simulink model "servotestin"  (R2020b)
settings: Solver=VariableStepAuto  StartTime=0.0  StopTime=10.0  RelTol=1e-3
model workspace (MAT data in the model file):
  BACKLASH_DEADBAND_RAD = Simulink.Parameter
  BACKLASH_DEADBAND_RAD.Value = 0.349065850399
  BACKLASH_DEADBAND_RAD.DataType = 'auto'
  BACKLASH_DEADBAND_RAD.Dimensions = [1 1]
  LEG_INERTIA = Simulink.Parameter
  LEG_INERTIA.Value = 0.01
  LEG_INERTIA.DataType = 'auto'
  LEG_INERTIA.Dimensions = [1 1]
libraries: fl_lib x7, nesl_utility x5, ee_lib x3, simulink_extras x2
settings Model: OrderedModelArguments=off  Creator=Adam  LastModifiedBy=Adam

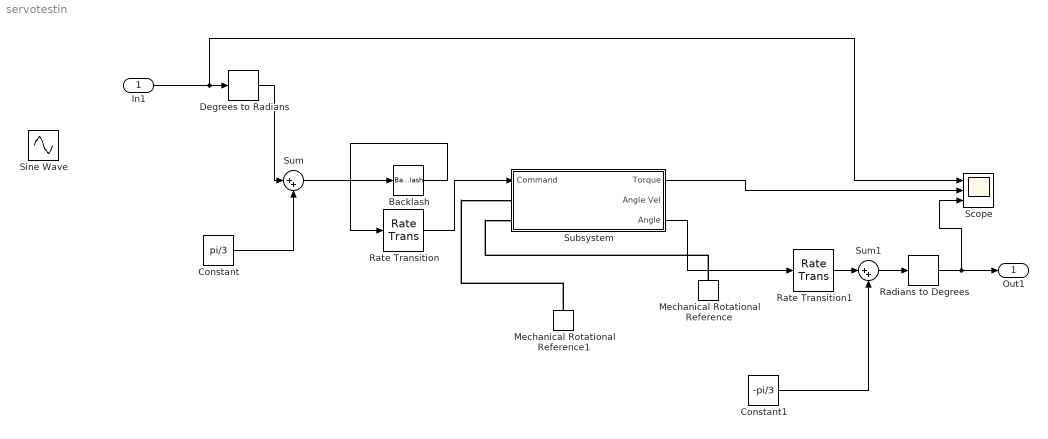
== system servotestin ==
  In1 : Inport
  Backlash : Backlash  BacklashWidth=BACKLASH_DEADBAND_RAD_M  InitialOutput=pi / 3
  Constant : Constant  Value=pi/3
  Constant1 : Constant  Value=-pi/3
  Degrees to Radians : simulink_extras/Transformations/Degrees to Radians
  Mechanical Rotational Reference : fl_lib/Mechanical/Rotational Elements/Mechanical Rotational Reference
  Mechanical Rotational Reference1 : fl_lib/Mechanical/Rotational Elements/Mechanical Rotational Reference
  Radians to Degrees : simulink_extras/Transformations/Radians to Degrees
  Rate Transition : RateTransition  InitialCondition=pi/3  OutPortSampleTime=1/330
  Rate Transition1 : RateTransition  InitialCondition=pi/3  OutPortSampleTime=.015
  Scope : Scope  NumInputPorts=3
  Sine Wave : Sin  Amplitude=20  Frequency=16  SampleTime=0
  Subsystem : Subsystem
  Sum : Sum  Inputs=|++
  Sum1 : Sum  Inputs=|++
  Out1 : Outport
  wires:
  In1/1 -> Scope/1, Degrees to Radians/1
  Subsystem/3(Angle) -> Rate Transition1/1
  Constant/1 -> Sum/2
  Sum/1 -> Backlash/1
  Rate Transition/1 -> Subsystem/1(Command)
  Subsystem/1(Torque) -> Scope/2
  Backlash/1 -> Rate Transition/1
  Degrees to Radians/1 -> Sum/1
  Radians to Degrees/1 -> Scope/3, Out1/1
  Constant1/1 -> Sum1/2
  Sum1/1 -> Radians to Degrees/1
  Rate Transition1/1 -> Sum1/1
  connections:
  Mechanical Rotational Reference1/LConn1 -- Subsystem/LConn1
  Mechanical Rotational Reference/LConn1 -- Subsystem/LConn2

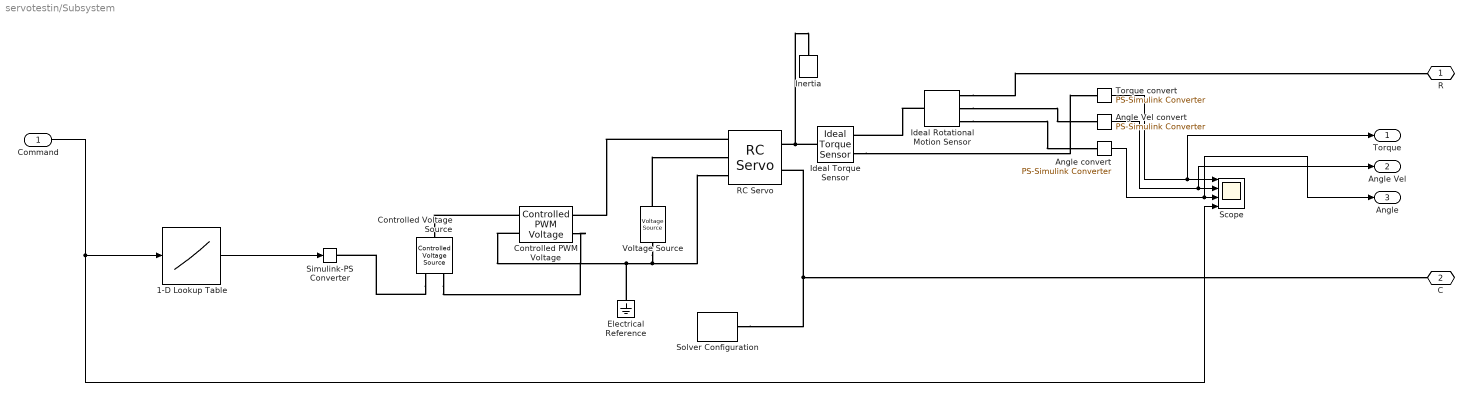
== system servotestin/Subsystem ==
  Command : Inport
  1-D Lookup Table : Lookup_n-D  NumberOfTableDimensions=1  BreakpointsForDimension1=[0 2*pi/3]  Table=[1.485 3.465]  InternalRulePriority=Speed  RndMeth=Simplest  InputSameDT=on
  Angle Vel convert : nesl_utility/PS-Simulink Converter  PhysicalDomain=network_engine_domain  SubClassName=ps_output  LeftPortType=input  RightPortType=output  PseudoPeriodic=off  Frequencies=[]  Unit=inherit  AffineConversion=off
  Angle convert : nesl_utility/PS-Simulink Converter  PhysicalDomain=network_engine_domain  SubClassName=ps_output  LeftPortType=input  RightPortType=output  PseudoPeriodic=off  Frequencies=[]  Unit=inherit  AffineConversion=off
  Controlled PWM Voltage : ee_lib/Integrated Circuits/Controlled PWM Voltage  F=330 Hz  TD=0 s  pulse_width_offset=0 s  pulse_min=0 s  Vmin=0 V  Vmax=5 V  Vm=5 V  pwm_or_av=1  event_type=1  sample_time=1e-6 s  u_min=0  u_max=1
  Controlled Voltage Source : fl_lib/Electrical/Electrical Sources/Controlled Voltage Source
  Electrical Reference : fl_lib/Electrical/Electrical Elements/Electrical Reference
  Ideal Rotational Motion Sensor : fl_lib/Mechanical/Mechanical Sensors/Ideal Rotational Motion Sensor  wrap_angle=simscape.enum.onoff.off  offset=60 deg
  Ideal Torque Sensor : fl_lib/Mechanical/Mechanical Sensors/Ideal Torque Sensor
  Inertia : fl_lib/Mechanical/Rotational Elements/Inertia  inertia=LEG_INERTIA_M kg*m^2  num_ports=foundation.enum.numPorts2.one  w_specify=off  w_priority=High  w=0 rad/s  w_nominal_specify=off  w_nominal_unit=rad/s  w_nominal_value=1  t_specify=off  t_priority=None  t=0 N*m  t_nominal_specify=off  t_nominal_unit=N*m  t_nominal_value=1
  RC Servo : ee_lib/Electromechanical/Brushed Motors/RC Servo  stall_torque=35 kg*cm  time_60=.11 s  nominal_voltage=7.2 V  rotational_range=[0, 120] deg  pulse_width_range=[900, 2100] us  threshold=3 V  R_s=18 kOhm  resolution=0.2 deg  angle_meas_error=0 deg  backdrive_torque=0.5 kg*cm  ratio=320  inertia=0.01 g*cm^2  endstop_angles=[-5, 185] deg  endstop_stiffness=1e6 N*m/rad  endstop_damping=0.01 N*m/(rad/s)  enable_faults=0  fault_action=1  fault_type=1  enable_temporal_fault=0  t_fault=1 s  enable_behavioral_fault=0  max_permissible_current=1 A  t_fail_on_current=1 s  angle_specify=on  angle_priority=High  angle=60 deg  angle_nominal_specify=off  angle_nominal_unit=deg  angle_nominal_value=1  w_specify=off  w_priority=High  w=0 deg/s  w_nominal_specify=off  w_nominal_unit=deg/s  w_nominal_value=1  torque_specify=off  torque_priority=None  torque=0 N*m  torque_nominal_specify=off  torque_nominal_unit=N*m  torque_nominal_value=1  pulse_width_specify=off  pulse_width_priority=Low  pulse_width=1.5 ms  i_specify=off  i_priority=None  i=0 A  i_nominal_specify=off  i_nominal_unit=A  i_nominal_value=1  i_s_specify=off  i_s_priority=None  i_s=0 A  i_s_nominal_specify=off  i_s_nominal_unit=A  i_s_nominal_value=1  motor_torque_specify=off  motor_torque_priority=None  motor_torque=0 N*m  motor_torque_nominal_specify=off  motor_torque_nominal_unit=N*m  motor_torque_nominal_value=1  power_dissipated_specify=off  power_dissipated_priority=None  power_dissipated=0 W  power_dissipated_nominal_specify=off  power_dissipated_nominal_unit=W  power_dissipated_nominal_value=1  angle_demand_specify=off  angle_demand_priority=None  angle_demand=90 deg  angle_demand_nominal_specify=off  angle_demand_nominal_unit=deg  angle_demand_nominal_value=1  faulted_specify=off  faulted_priority=None  faulted=0  faulted_nominal_specify=off  faulted_nominal_unit=1  faulted_nominal_value=1
      settings: SourceProductBaseCode=PS  InternalSimscapePortConfiguration="{\"Bottom\":[],\"Left\":[{\"id\":\"s\",\"label\":\"s\",\"type\":\"foundation.electrical.electrical\"},{\"id\":\"p\",\"label\":\"+\",\"type\":\"foundation.electrical.electrical\"},{\"id\":\"n\",\"label\":\"-\",\"type\":\"foundation.electrical.electrical\"}],\"Right\":[{\"id\":\"R\",\"label\":\"R\",\"type\":\"foundation.mechanical.rotational.rotational\"},{\"id\":\"C\",\"label\":\"C\",\"type\":\"foundation.mechanical.rotational.rotational\"}],\"Top\":[]}"
  Scope : Scope  NumInputPorts=4
  Simulink-PS Converter : nesl_utility/Simulink-PS Converter  PhysicalDomain=network_engine_domain  SubClassName=ps_input  LeftPortType=input  RightPortType=output  PseudoPeriodic=off  Frequencies=[]  NoiseDistribution=none  NoiseParameters=[]  Unit=V  AffineConversion=off  FilteringAndDerivatives=provide  SimscapeFilterOrder=1  InputFilterTimeConstant=0.001  UdotUserProvided=0
  Solver Configuration : nesl_utility/Solver Configuration  PhysicalDomain=network_engine_domain  SubClassName=solver  LeftPortType=input  RightPortType=generic  Tones=[]  Harmonics=[]  SimulateNoise=off  Profile=off  UseLocalSampling=off  EnableSwitchedLinearOptims=on  FrequencyDomain=off  UseCCode=off  RelTol=0.001  AbsTol=1e-06  MinStep=1e-09  ToWorkspace=off  RevertToSquareIcSolve=off  NumHomotopyIterations=100  PhasorMode=off  PhasorModeNumHarmonics=1  DoDC=off  ResidualTolerance=1e-09  UseLocalSolver=off  LocalSolverChoice=NE_BACKWARD_EULER_ADVANCER  LocalSolverSampleTime=0.001  DoFixedCost=off  MaxNonlinIter=3  MaxModeIter=2  ComputeImpulses=off  ImpulseIterations=2  LinearAlgebra=auto  EquationFormulation=NE_TIME_EF  DelaysMemoryBudget=1024  AutomaticFiltering=on  FilteringTimeConstant=0.001  PartitionStorageMethod=AS_NEEDED  PartitionMemoryBudget=1024  PartitionMethod=ROBUST
  Torque convert : nesl_utility/PS-Simulink Converter  PhysicalDomain=network_engine_domain  SubClassName=ps_output  LeftPortType=input  RightPortType=output  PseudoPeriodic=off  Frequencies=[]  Unit=inherit  AffineConversion=off
  Voltage Source : ee_lib/Sources/Voltage Source  dc_voltage=7.1 V  ac_voltage=0 V  ac_shift=0 rad  ac_frequency=60 Hz  noise_mode=0  PSD=0 V^2/Hz  repeatability=1  auto_seed=4205327602  user_seed=0  sample_time=1e-3 s  i_specify=off  i_priority=None  i=0 A  i_nominal_specify=off  i_nominal_unit=A  i_nominal_value=1  v_specify=off  v_priority=None  v=0 V  v_nominal_specify=off  v_nominal_unit=V  v_nominal_value=1
  R : PMIOPort  Side=Left
  C : PMIOPort  Port=2  Side=Left
  Torque : Outport
  Angle Vel : Outport  Port=2
  Angle : Outport  Port=3
  wires:
  Angle convert/1 -> Angle/1, Scope/3
  1-D Lookup Table/1 -> Simulink-PS Converter/1
  Command/1 -> 1-D Lookup Table/1, Scope/4
  Torque convert/1 -> Torque/1, Scope/1
  Angle Vel convert/1 -> Angle Vel/1, Scope/2
  connections:
  Voltage Source/RConn1 -- Electrical Reference/LConn1 -- Controlled Voltage Source/RConn2 -- Controlled PWM Voltage/RConn2 -- Controlled PWM Voltage/LConn2 -- RC Servo/LConn3
  Controlled Voltage Source/RConn1 -- Simulink-PS Converter/RConn1
  Ideal Torque Sensor/LConn1 -- Inertia/LConn1 -- RC Servo/RConn1
  Controlled PWM Voltage/LConn1 -- Controlled Voltage Source/LConn1
  Solver Configuration/RConn1 -- C/RConn1 -- RC Servo/RConn2
  RC Servo/LConn1 -- Controlled PWM Voltage/RConn1
  Ideal Rotational Motion Sensor/RConn2 -- Angle Vel convert/LConn1
  Ideal Rotational Motion Sensor/LConn1 -- Ideal Torque Sensor/RConn1
  Ideal Torque Sensor/RConn2 -- Torque convert/LConn1
  Ideal Rotational Motion Sensor/RConn3 -- Angle convert/LConn1
  Voltage Source/LConn1 -- RC Servo/LConn2
  Ideal Rotational Motion Sensor/RConn1 -- R/RConn1
